simulink model "untitled2"  (R2021a)
settings: Solver=FixedStepAuto  StartTime=0.0  StopTime=31  RelTol=1e-3
libraries: simulink_extras x6, simulink x5, hdlsllib x1
settings Model: Creator=PS  LastModifiedBy=PS

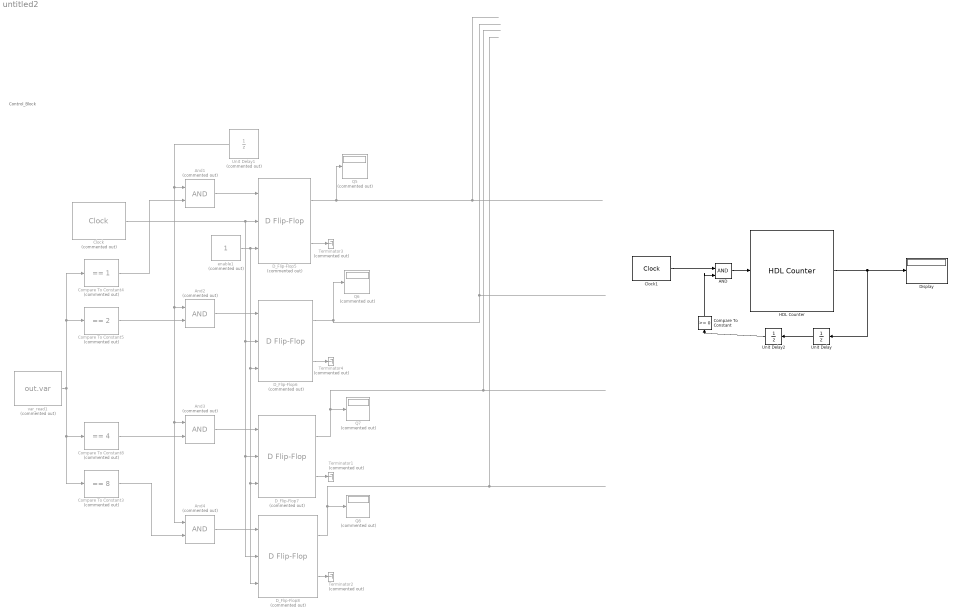
== system untitled2 ==
  note: Control_Block
  AND : Logic  IconShape=distinctive  AllPortsSameDT=off  OutDataTypeStr=boolean
  And{1..4} (4 alike) : Logic  Commented=on  IconShape=distinctive  AllPortsSameDT=off  OutDataTypeStr=boolean
  Clock : simulink_extras/Flip Flops/Clock  Commented=on  period=1
  Clock1 : simulink_extras/Flip Flops/Clock  period=1
  Compare To Constant : simulink/Logic and Bit Operations/Compare To Constant  relop=>=  const=0  OutDataTypeStr=boolean
  Compare To Constant3 : simulink/Logic and Bit Operations/Compare To Constant  Commented=on  relop===  const=8  OutDataTypeStr=boolean
  Compare To Constant4 : simulink/Logic and Bit Operations/Compare To Constant  Commented=on  relop===  const=1  OutDataTypeStr=boolean
  Compare To Constant5 : simulink/Logic and Bit Operations/Compare To Constant  Commented=on  relop===  const=2  OutDataTypeStr=boolean
  Compare To Constant8 : simulink/Logic and Bit Operations/Compare To Constant  Commented=on  relop===  const=4  OutDataTypeStr=boolean
  D_Flip-Flop{5..8} (4 alike) : simulink_extras/Flip Flops/D Flip-Flop  Commented=on
  Display : Display
  HDL Counter : hdlsllib/Sources/HDL Counter  CountType=Count limited  CountInit=0  CountStep=1  CountMax=10  CountFromType=Initial value  CountFrom=0  CountResetPort=off  CountLoadPort=off  CountEnbPort=on  CountDirPort=off  CountHitOutputPort=off  CountDataType=Unsigned  CountWordLen=8  CountFracLen=0  CountSampTime=1
  Q{5..8} (4 alike) : Display  Commented=on
  Terminator{1..4} (4 alike) : Terminator  Commented=on
  Unit Delay : UnitDelay  SampleTime=-1  HasFrameUpgradeWarning=on
  Unit Delay1 : UnitDelay  Commented=on  SampleTime=-1  HasFrameUpgradeWarning=on
  Unit Delay2 : UnitDelay  SampleTime=-1  HasFrameUpgradeWarning=on
  enable1 : Constant  Commented=on  OutDataTypeStr=boolean
  var_read1 : FromWorkspace  Commented=on  VariableName=out.var
  wires:
  Unit Delay1/1 -> And1/1, And4/1, And3/1, And2/1
  enable1/1 -> D_Flip-Flop8/3, D_Flip-Flop7/3, D_Flip-Flop6/3, D_Flip-Flop5/3
  D_Flip-Flop5/2 -> Terminator3/1
  D_Flip-Flop8/2 -> Terminator2/1
  D_Flip-Flop6/2 -> Terminator4/1
  D_Flip-Flop6/1 -> Q6/1
  D_Flip-Flop7/2 -> Terminator1/1
  D_Flip-Flop8/1 -> Q8/1
  D_Flip-Flop5/1 -> Q5/1
  var_read1/1 -> Compare To Constant4/1, Compare To Constant5/1, Compare To Constant3/1, Compare To Constant8/1
  D_Flip-Flop7/1 -> Q7/1
  Compare To Constant5/1 -> And2/2
  And1/1 -> D_Flip-Flop5/1
  Compare To Constant4/1 -> And1/2
  Clock/1 -> D_Flip-Flop5/2, D_Flip-Flop8/2, D_Flip-Flop7/2, D_Flip-Flop6/2
  And2/1 -> D_Flip-Flop6/1
  And3/1 -> D_Flip-Flop7/1
  Compare To Constant8/1 -> And3/2
  And4/1 -> D_Flip-Flop8/1
  Compare To Constant3/1 -> And4/2
  HDL Counter/1 -> Unit Delay/1, Display/1
  Unit Delay2/1 -> Compare To Constant/1
  AND/1 -> HDL Counter/1
  Clock1/1 -> AND/1
  Compare To Constant/1 -> AND/2
  Unit Delay/1 -> Unit Delay2/1
